simulink model "LQR_Test"  (R2019a)
settings: Solver=VariableStepAuto  StartTime=0  StopTime=10  FixedStep=tStep  RelTol=1e-3  EnableMultiTasking=on
values from neighbouring files (symbols this model uses):
  A = [0 1 0 0 0 0;9.84 -0.33 -6.9 0.08 -10.85 0;0 0 0 1 0 0;-115.14 -0.01 -0.28 -0.83 108.56 0;0 0 0 0 0 1;-770.27 1e-16 2*10^-15 -5.55 792.07 0]    [LQR_PWERT.m]
  B = [0; -42.95; 0; 429.59; 0; 2931.20]    [LQR_PWERT.m]
  K_LQR = lqr(A,B,Q,R)    [LQR_PWERT.m]
  x0 = [-pi/6 0 0.2 0 0 0]    [LQR_PWERT.m]
settings Model: Creator=loehning  LastModifiedBy=quynh
settings DataIOCC: SaveFormat=Array  SignalLoggingSaveFormat=ModelDataLogs  ReturnWorkspaceOutputs=off
settings OptimizationCC: ExpressionDepthLimit=2147483647  LifeSpan=inf
settings DebuggingCC: UnderspecifiedInitializationDetection=Classic  MergeDetectMultiDrivingBlocksExec=none  SolverPrmCheckMsg=warning  FcnCallInpInsideContextMsg=warning  StateNameClashWarn=warning  PregeneratedLibrarySubsystemCodeDiagnostic=none  SFUnexpectedBacktrackingDiag=warning  SFNoUnconditionalDefaultTransitionDiag=warning  SFExecutionAtInitializationDiag=none  ArithmeticOperatorsInVariantConditions=warning
settings HardwareCC: ProdBitPerPointer=32  ProdBitPerSizeT=32  ProdBitPerPtrDiffT=32  ProdLargestAtomicFloat=None  ProdIntDivRoundTo=Undefined  ProdEndianess=Unspecified  ProdWordSize=32  ProdHWDeviceType=32-bit Generic
settings ModelReferenceCC: PropagateSignalLabelsOutOfModel=off
settings SFSimCC: SimUseLocalCustomCode=off
settings RTWCC: RTWUseLocalCustomCode=off
settings CodeAppCC: StateflowObjectComments=on
settings GRTTargetCC: TargetLangStandard=C89/C90 (ANSI)  GeneratePreprocessorConditionals=Disable all  CombineOutputUpdateFcns=off  GRTInterface=on
settings ConfigComp: CovMetricSettings=dw  CovHtmlReporting=on  CovSaveCumulativeToWorkspaceVar=on  CovSaveSingleToWorkspaceVar=on  CovExternalEMLEnable=off  CovSFcnEnable=off

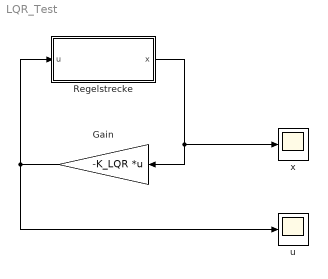
== system LQR_Test ==
  Gain : Gain  Gain=-K_LQR  Multiplication=Matrix(K*u)
  "Regelstrecke " : Subsystem
  u : Scope
  x : Scope
  wires:
  "Regelstrecke "/1(x) -> Gain/1, x/1
  Gain/1 -> u/1, "Regelstrecke "/1(u)

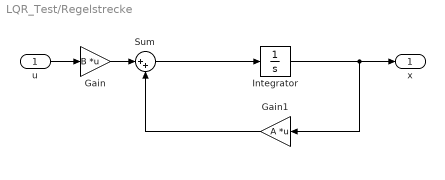
== system LQR_Test/Regelstrecke  ==
  u : Inport
  Gain : Gain  Gain=B  Multiplication=Matrix(K*u)
  Gain1 : Gain  Gain=A  Multiplication=Matrix(K*u)
  Integrator : Integrator  InitialCondition=x0
  Sum : Sum  Inputs=|++
  x : Outport
  wires:
  Integrator/1 -> Gain1/1, x/1
  Gain/1 -> Sum/1
  u/1 -> Gain/1
  Sum/1 -> Integrator/1
  Gain1/1 -> Sum/2
